simulink model "vitis_hls"  (R2021a)
settings: Solver=VariableStepAuto  StartTime=0.0  StopTime=1000  RelTol=1e-3
undefined symbols (not defined in the file or in its folder): AXI4, Lite
libraries: hdlBasic x77, xbsIndex_r4 x1
settings Model: Creator=sl186  LastModifiedBy=sl186

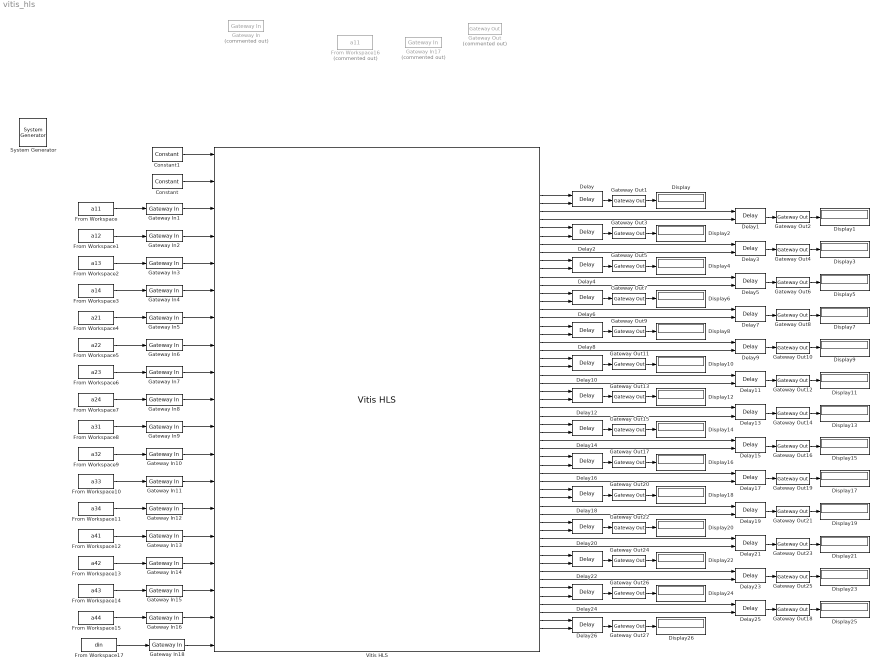
== system vitis_hls ==
  " System Generator" : xbsIndex_r4/ System Generator  Tag=genX  xilinxfamily=zynq  part=xc7z020  speed=-1  package=clg484  synthesis_tool=Vivado  clock_wrapper=Clock Enables  directory=./netlist  proj_type=Vivado  Synth_file=Vivado Synthesis Defaults  Impl_file=Vivado Implementation Defaults  testbench=off  simulink_period=1  sysclk_period=10  dcm_input_clock_period=10  incr_netlist=off  trim_vbits=Everywhere in SubSystem  dbl_ovrd=According to Block Masks  core_generation=According to Block Masks  run_coregen=off  deprecated_control=off  eval_field=0  block_type=sysgen
  Constant : hdlBasic/Constant  const=1  gui_display_data_type=Boolean  arith_type=Boolean  n_bits=16  bin_pt=14  preci_type=Single  exp_width=8  frac_width=24  explicit_period=off  period=1  XmcBlockStatus=1  maskContainerNames=tabcontainer1  block_type=constant  block_config=sysgen:Constant_config
  Constant1 : hdlBasic/Constant  const=0  gui_display_data_type=Boolean  arith_type=Boolean  n_bits=16  bin_pt=14  preci_type=Single  exp_width=8  frac_width=24  explicit_period=off  period=1  XmcBlockStatus=1  maskContainerNames=tabcontainer1  block_type=constant  block_config=sysgen:Constant_config
  Delay{,1..26} (27 alike) : hdlBasic/Delay  rst=off  en=on  latency=1  reg_retiming=off  XmcBlockStatus=1  maskContainerNames=group1  block_type=delay  block_config=sysgen:Delay_config
  Display{,1..26} (27 alike) : Display
  From Workspace : FromWorkspace  VariableName=a11  OutputAfterFinalValue=Holding final value
  From Workspace1 : FromWorkspace  VariableName=a12  OutputAfterFinalValue=Holding final value
  From Workspace10 : FromWorkspace  VariableName=a33  OutputAfterFinalValue=Holding final value
  From Workspace11 : FromWorkspace  VariableName=a34  OutputAfterFinalValue=Holding final value
  From Workspace12 : FromWorkspace  VariableName=a41  OutputAfterFinalValue=Holding final value
  From Workspace13 : FromWorkspace  VariableName=a42  OutputAfterFinalValue=Holding final value
  From Workspace14 : FromWorkspace  VariableName=a43  OutputAfterFinalValue=Holding final value
  From Workspace15 : FromWorkspace  VariableName=a44  OutputAfterFinalValue=Holding final value
  From Workspace16 : FromWorkspace  Commented=on  VariableName=a11
  From Workspace17 : FromWorkspace  VariableName=din
  From Workspace2 : FromWorkspace  VariableName=a13  OutputAfterFinalValue=Holding final value
  From Workspace3 : FromWorkspace  VariableName=a14  OutputAfterFinalValue=Holding final value
  From Workspace4 : FromWorkspace  VariableName=a21  OutputAfterFinalValue=Holding final value
  From Workspace5 : FromWorkspace  VariableName=a22  OutputAfterFinalValue=Holding final value
  From Workspace6 : FromWorkspace  VariableName=a23  OutputAfterFinalValue=Holding final value
  From Workspace7 : FromWorkspace  VariableName=a24  OutputAfterFinalValue=Holding final value
  From Workspace8 : FromWorkspace  VariableName=a31  OutputAfterFinalValue=Holding final value
  From Workspace9 : FromWorkspace  VariableName=a32  OutputAfterFinalValue=Holding final value
  Gateway In : hdlBasic/Gateway In  Commented=on  gui_display_data_type=Fixed-point  arith_type=Signed (2's comp)  n_bits=16  bin_pt=14  preci_type=Single  exp_width=8  frac_width=24  rows=1  columns=1  quantization="Round  (unbiased: +/- Inf)"  overflow=Saturate  period=1  UseAsADC=off  ADCChannel='1'  interface=None  automatic_assignment=on  address_offset=hex2dec('00')  intf_name=''  intf_description=''  default_value=0  timing_constraint=None  locs_specified=off  LOCs={}  io_standard={}  inherit_from_input=off  hdl_port=on  XmcBlockStatus=1  maskContainerNames=group4  block_type=gatewayin  block_config=sysgen:gateway_in_config  block_width_w=590  block_height_w=620  block_width=640  block_height=850
  Gateway In{1..16,18} (17 alike) : hdlBasic/Gateway In  gui_display_data_type=Fixed-point  arith_type=Signed (2's comp)  n_bits=24  bin_pt=16  preci_type=Single  exp_width=8  frac_width=24  rows=1  columns=1  quantization="Round  (unbiased: +/- Inf)"  overflow=Saturate  period=1  UseAsADC=off  ADCChannel='1'  interface=AXI4-Lite  automatic_assignment=on  address_offset=hex2dec('00')  intf_name=''  intf_description=''  default_value=0  timing_constraint=None  locs_specified=off  LOCs={}  io_standard={}  inherit_from_input=off  hdl_port=on  XmcBlockStatus=1  maskContainerNames=group4  block_type=gatewayin  block_config=sysgen:gateway_in_config  block_width_w=590  block_height_w=620  block_width=640  block_height=850
  Gateway In17 : hdlBasic/Gateway In  Commented=on  gui_display_data_type=Fixed-point  arith_type=Signed (2's comp)  n_bits=24  bin_pt=16  preci_type=Single  exp_width=8  frac_width=24  rows=1  columns=1  quantization="Round  (unbiased: +/- Inf)"  overflow=Saturate  period=1  UseAsADC=off  ADCChannel='1'  interface=AXI4-Lite  automatic_assignment=on  address_offset=hex2dec('00')  intf_name=''  intf_description=''  default_value=0  timing_constraint=None  locs_specified=off  LOCs={}  io_standard={}  inherit_from_input=off  hdl_port=on  XmcBlockStatus=1  maskContainerNames=group4  block_type=gatewayin  block_config=sysgen:gateway_in_config  block_width_w=590  block_height_w=620  block_width=640  block_height=850
  Gateway Out : hdlBasic/Gateway Out  Commented=on  inherit_from_input=off  hdl_port=on  rows=1  columns=1  UseAsDAC=off  DACChannel='1'  interface=None  automatic_assignment=on  address_offset=hex2dec('00')  intf_name=''  intf_description=''  timing_constraint=None  locs_specified=off  LOCs={}  io_standard={}  XmcBlockStatus=1  maskContainerNames=group4  block_type=gatewayout  block_config=sysgen:gateway_out_config  block_width_w=590  block_height_w=620  block_width=620  block_height=750
  Gateway Out{1..27} (27 alike) : hdlBasic/Gateway Out  inherit_from_input=off  hdl_port=on  rows=1  columns=1  UseAsDAC=off  DACChannel='1'  interface=AXI4-Lite  automatic_assignment=on  address_offset=hex2dec('00')  intf_name=''  intf_description=''  timing_constraint=None  locs_specified=off  LOCs={}  io_standard={}  XmcBlockStatus=1  maskContainerNames=group4  block_type=gatewayout  block_config=sysgen:gateway_out_config  block_width_w=590  block_height_w=620  block_width=620  block_height=750
  Vitis HLS : hdlBasic/Vitis HLS  anytable='C:\ELEC522\sl186\Assignment5V3\A5V3FIX\solution1'  fast_sim=off  display_datatype=off  rate_propagation_method=Simulink system period  model_file_path=''  latency=1  block_type=vitis_hls
      settings: infoedit=This block allows including C,C++ and SystemC source files in System Generator for DSP designs.
  wires:
  From Workspace/1 -> Gateway In1/1
  From Workspace1/1 -> Gateway In2/1
  From Workspace2/1 -> Gateway In3/1
  From Workspace3/1 -> Gateway In4/1
  From Workspace5/1 -> Gateway In6/1
  From Workspace4/1 -> Gateway In5/1
  From Workspace6/1 -> Gateway In7/1
  From Workspace7/1 -> Gateway In8/1
  From Workspace12/1 -> Gateway In13/1
  From Workspace11/1 -> Gateway In12/1
  From Workspace8/1 -> Gateway In9/1
  From Workspace13/1 -> Gateway In14/1
  From Workspace10/1 -> Gateway In11/1
  From Workspace15/1 -> Gateway In16/1
  From Workspace9/1 -> Gateway In10/1
  From Workspace14/1 -> Gateway In15/1
  Gateway In1/1 -> Vitis HLS/3
  Gateway In2/1 -> Vitis HLS/4
  Gateway In16/1 -> Vitis HLS/18
  Gateway In3/1 -> Vitis HLS/5
  Gateway In4/1 -> Vitis HLS/6
  Gateway In5/1 -> Vitis HLS/7
  Gateway In6/1 -> Vitis HLS/8
  Gateway In7/1 -> Vitis HLS/9
  Gateway In8/1 -> Vitis HLS/10
  Gateway In9/1 -> Vitis HLS/11
  Gateway In10/1 -> Vitis HLS/12
  Gateway In11/1 -> Vitis HLS/13
  Gateway In12/1 -> Vitis HLS/14
  Gateway In13/1 -> Vitis HLS/15
  Gateway In14/1 -> Vitis HLS/16
  Gateway In15/1 -> Vitis HLS/17
  Vitis HLS/5 -> Delay/2
  Vitis HLS/4 -> Delay/1
  Delay/1 -> Gateway Out1/1
  Gateway Out1/1 -> Display/1
  Delay1/1 -> Gateway Out2/1
  Gateway Out2/1 -> Display1/1
  Vitis HLS/6 -> Delay1/1
  Vitis HLS/7 -> Delay1/2
  Gateway Out3/1 -> Display2/1
  Delay3/1 -> Gateway Out4/1
  Gateway Out4/1 -> Display3/1
  Vitis HLS/11 -> Delay3/2
  Vitis HLS/10 -> Delay3/1
  Delay2/1 -> Gateway Out3/1
  Vitis HLS/8 -> Delay2/1
  Vitis HLS/9 -> Delay2/2
  Vitis HLS/13 -> Delay4/2
  Vitis HLS/17 -> Delay6/2
  Delay4/1 -> Gateway Out5/1
  Vitis HLS/12 -> Delay4/1
  Vitis HLS/15 -> Delay5/2
  Vitis HLS/19 -> Delay7/2
  Vitis HLS/18 -> Delay7/1
  Delay6/1 -> Gateway Out7/1
  Gateway Out7/1 -> Display6/1
  Vitis HLS/16 -> Delay6/1
  Gateway Out5/1 -> Display4/1
  Delay7/1 -> Gateway Out8/1
  Delay5/1 -> Gateway Out6/1
  Gateway Out6/1 -> Display5/1
  Gateway Out8/1 -> Display7/1
  Vitis HLS/14 -> Delay5/1
  Delay8/1 -> Gateway Out9/1
  Vitis HLS/20 -> Delay8/1
  Vitis HLS/23 -> Delay9/2
  Vitis HLS/27 -> Delay11/2
  Vitis HLS/26 -> Delay11/1
  Delay10/1 -> Gateway Out11/1
  Gateway Out14/1 -> Display13/1
  Gateway Out16/1 -> Display15/1
  Delay15/1 -> Gateway Out16/1
  Gateway Out11/1 -> Display10/1
  Delay13/1 -> Gateway Out14/1
  Gateway Out13/1 -> Display12/1
  Delay11/1 -> Gateway Out12/1
  Gateway Out12/1 -> Display11/1
  Gateway Out15/1 -> Display14/1
  Delay14/1 -> Gateway Out15/1
  Vitis HLS/24 -> Delay10/1
  Vitis HLS/28 -> Delay12/1
  Vitis HLS/34 -> Delay15/1
  Vitis HLS/30 -> Delay13/1
  Vitis HLS/33 -> Delay14/2
  Vitis HLS/21 -> Delay8/2
  Vitis HLS/25 -> Delay10/2
  Vitis HLS/29 -> Delay12/2
  Vitis HLS/31 -> Delay13/2
  Vitis HLS/32 -> Delay14/1
  Gateway Out9/1 -> Display8/1
  Delay9/1 -> Gateway Out10/1
  Vitis HLS/35 -> Delay15/2
  Gateway Out10/1 -> Display9/1
  Vitis HLS/22 -> Delay9/1
  Delay12/1 -> Gateway Out13/1
  Gateway Out18/1 -> Display25/1
  Gateway Out26/1 -> Display24/1
  Delay16/1 -> Gateway Out17/1
  Vitis HLS/36 -> Delay16/1
  Vitis HLS/39 -> Delay17/2
  Vitis HLS/43 -> Delay19/2
  Vitis HLS/42 -> Delay19/1
  Delay25/1 -> Gateway Out18/1
  Delay18/1 -> Gateway Out20/1
  Gateway Out23/1 -> Display21/1
  Delay24/1 -> Gateway Out26/1
  Gateway Out25/1 -> Display23/1
  Delay23/1 -> Gateway Out25/1
  Gateway Out20/1 -> Display18/1
  Delay21/1 -> Gateway Out23/1
  Gateway Out22/1 -> Display20/1
  Delay19/1 -> Gateway Out21/1
  Gateway Out21/1 -> Display19/1
  Gateway Out24/1 -> Display22/1
  Delay22/1 -> Gateway Out24/1
  Vitis HLS/40 -> Delay18/1
  Vitis HLS/52 -> Delay24/1
  Vitis HLS/54 -> Delay25/1
  Vitis HLS/53 -> Delay24/2
  Vitis HLS/44 -> Delay20/1
  Vitis HLS/50 -> Delay23/1
  Vitis HLS/46 -> Delay21/1
  Vitis HLS/49 -> Delay22/2
  Vitis HLS/37 -> Delay16/2
  Vitis HLS/41 -> Delay18/2
  Vitis HLS/45 -> Delay20/2
  Vitis HLS/47 -> Delay21/2
  Vitis HLS/48 -> Delay22/1
  Gateway Out17/1 -> Display16/1
  Delay17/1 -> Gateway Out19/1
  Vitis HLS/55 -> Delay25/2
  Vitis HLS/51 -> Delay23/2
  Gateway Out19/1 -> Display17/1
  Vitis HLS/38 -> Delay17/1
  Delay20/1 -> Gateway Out22/1
  Constant/1 -> Vitis HLS/2
  Constant1/1 -> Vitis HLS/1
  From Workspace17/1 -> Gateway In18/1
  Gateway In18/1 -> Vitis HLS/19
  Vitis HLS/57 -> Delay26/2
  Delay26/1 -> Gateway Out27/1
  Gateway Out27/1 -> Display26/1
  Vitis HLS/56 -> Delay26/1
